simulink model "AC_Quadcopter_Simulation"  (R2019b)
settings: Solver=ode45  StartTime=0  StopTime=10  FixedStep=0.02  MaxStep=0.06  RelTol=1e-3  EnableMultiTasking=on
model workspace (MAT data in the model file):
  Sig = Simulink.Signal
  Sig.DataType = 'auto'
  Sig.Dimensions = -1
  Sig.DimensionsMode = 'auto'
  Sig.Complexity = 'auto'
  Sig.SampleTime = -1
  Sig.SamplingMode = 'auto'
undefined symbols (not defined in the file): IC, quadModel
libraries: simulink x4
Description:
  | This is a configurable quadcopter simulation.
  | This Simulink model demonstates attitude control.
  | 
  | Additional quadcopter modeling and simulation materials available at:
  | github.com/dch33/Quad-Sim
  | 
  | Copyright (C) 2014 D. Hartman, K. Landis, S. Moreno, J. Kim, M. Mehrer
  | 
  | License:
  |     This program is free software: you can redistribute it and/or modify
  |     it under the terms of the GNU LESSER GENERAL PUBLIC LICENSE as published by
  |     the Free Software Foundation, either version 3 of the License, or
  |     (at your option) any later version.
  | 
  |     This program is distributed in the hope that it will be useful,
  |     but WITHOUT ANY WARRANTY; without even the implied warranty of
  |     MERCHANTABILITY or FITNESS FOR A PARTICULAR PURPOSE.  See the
  |     GNU General Public License for more details.
  | 
  |     You should have received a copy of the GNU LESSER GENERAL PUBLIC LICENSE
  |     along with this program.  If not, see <http://www.gnu.org/licenses/>.
settings Model: ModifiedComment=davidhartman -- Fri Jun 06 23:19:51 2014 -- Version 1.5  Creator=David Hartman  LastModifiedBy=bhisma
settings Model: ModifiedHistory=|
  | davidhartman -- Fri Jun 06 23:19:51 2014 -- Version 1.5
  | 
  | 
  | davidhartman -- Fri Jun 06 23:19:51 2014 -- Version 1.5
  | 
  | 
  | davidhartman -- Fri Jun 06 22:53:10 2014 -- Version 1.3
settings SolverCC: AutoInsertRateTranBlk=on
settings DataIOCC: SaveFormat=Array  SignalLogging=off  ReturnWorkspaceOutputs=off
settings OptimizationCC: DefaultParameterBehavior=Inlined  LifeSpan=inf
settings DebuggingCC: UnderspecifiedInitializationDetection=Classic  MergeDetectMultiDrivingBlocksExec=none  SolverPrmCheckMsg=warning  UniqueDataStoreMsg=warning  StateNameClashWarn=warning  StrictBusMsg=WarnOnBusTreatedAsVector  SFUnexpectedBacktrackingDiag=warning  SFNoUnconditionalDefaultTransitionDiag=warning  SFExecutionAtInitializationDiag=none  ArithmeticOperatorsInVariantConditions=warning
settings HardwareCC: ProdBitPerPointer=32  ProdBitPerSizeT=32  ProdBitPerPtrDiffT=32  ProdLargestAtomicFloat=None  ProdIntDivRoundTo=Undefined  ProdEndianess=Unspecified  ProdWordSize=32  ProdHWDeviceType=32-bit Generic
settings ModelReferenceCC: PropagateSignalLabelsOutOfModel=off
settings SFSimCC: SimUseLocalCustomCode=off  CustomCodeUndefinedFunction=UseInterfaceOnly
settings RTWCC: RTWUseLocalCustomCode=off
settings CodeAppCC: StateflowObjectComments=on
settings GRTTargetCC: TargetLangStandard=C89/C90 (ANSI)  GeneratePreprocessorConditionals=Disable all
settings ConfigComp: CovMetricSettings=dw  CovHtmlReporting=on  CovSaveCumulativeToWorkspaceVar=on  CovSaveSingleToWorkspaceVar=on  CovExternalEMLEnable=off

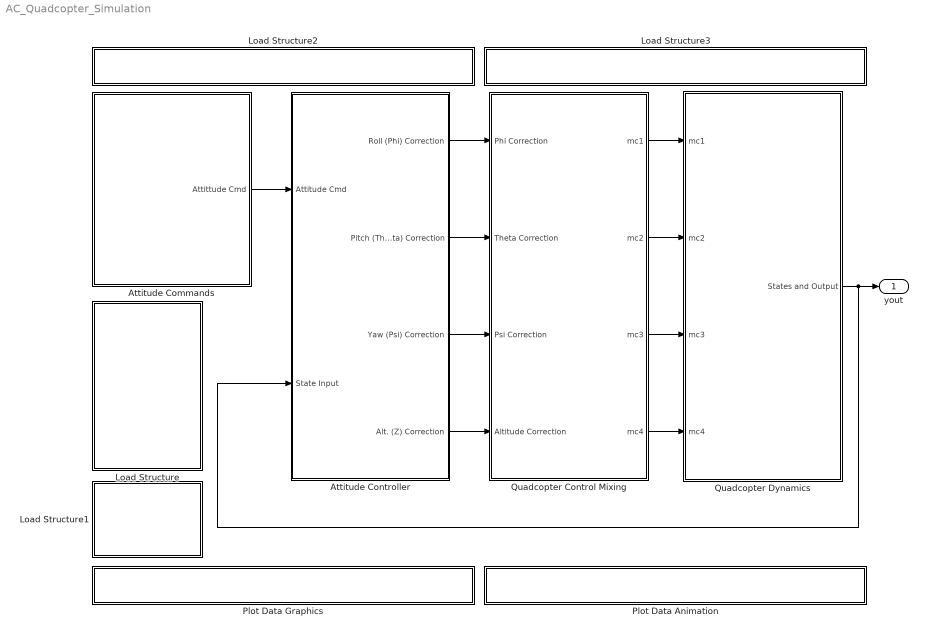
== system AC_Quadcopter_Simulation ==
  Attitude Commands : Subsystem
  Attitude Controller : Subsystem
  Load Structure : Subsystem
      settings: OpenFcn=|
      | uiopen('load')
      | if (exist('IC')==1 && exist('quadModel')==1)
      | set_param(bdroot, 'SimulationCommand', 'update')
      | end
      mask Display: fprintf('LOAD:\nQuadcopter\nModel Or\nInitial\nConditions');
  Load Structure1 : Subsystem
      settings: OpenFcn=|
      | if (exist('IC')==1 && exist('quadModel')==1 && exist('yout') && exist('tout'))
      | saveSimResults()
      | else
      | msgbox('No Data To Save!')
      | end
      mask Display: fprintf('SAVE:\nSimulation\nResults');
  Load Structure2 : Subsystem
      settings: OpenFcn=|
      | if exist('GUI_Modeling') == 2,
      | run('GUI_Modeling')
      | 
      | else
      | 
      | msgbox('The desired GUI must be first added to MATLABs path.')
      | 
      | end
      mask Display: fprintf('OPEN GUI: Build New \n Model');
  Load Structure3 : Subsystem
      settings: OpenFcn=|
      | if exist('GUI_IC') == 2,
      | run('GUI_IC')
      | 
      | else
      | 
      | msgbox('The desired GUI must be first added to MATLABs path.')
      | 
      | end
      mask Display: fprintf('OPEN GUI: Create Initial \n Conditions');
  Plot Data Animation : Subsystem
      settings: OpenFcn=|
      | if exist('QuadAnim4') == 2,
      |     if exist('yout')
      | 	run('QuadAnim4');
      |     else
      |     msgbox('Simulation must be run before data can be plotted.');
      |     end
      | else                                                                          msgbox('The desired GUI must be first added to MATLABs path.')
      | end
      mask Display: fprintf('OPEN GUI: Flight Animation')
  Plot Data Graphics : Subsystem
      settings: OpenFcn=|
      | if exist('yout')
      | yout = evalin('base', 'yout');
      | tout = evalin('base', 'tout');
      | quadPlots(yout, tout)
      | else
      | msgbox('Simulation must be run before data can be plotted.')
      | end
      mask Display: fprintf('OPEN PLOT: State Data')
  Quadcopter Control Mixing : Subsystem
      mask Display:
      | modelLoaded = evalin('base','exist(''quadModel'',''var'')');
      | if (modelLoaded==1)
      |     if (evalin('base','quadModel.plusConfig'))
      |     fprintf([' \n' ' \n'  'Configuration "+"']);
      |     else if (~evalin('base','quadModel.plusConfig'))
      |         fprintf([' \n' ' \n' 'Configuration "X"']);
      |         end
      |     end
      | else
      |     fprintf([' \n' ' \n'  'Model Not Loaded']);
      | end
  Quadcopter Dynamics : Subsystem
  yout : Outport
  wires:
  Quadcopter Dynamics/1(States and Output) -> yout/1, Attitude Controller/2(State Input)
  Quadcopter Control Mixing/1(mc1) -> Quadcopter Dynamics/1(mc1)
  Quadcopter Control Mixing/2(mc2) -> Quadcopter Dynamics/2(mc2)
  Quadcopter Control Mixing/3(mc3) -> Quadcopter Dynamics/3(mc3)
  Quadcopter Control Mixing/4(mc4) -> Quadcopter Dynamics/4(mc4)
  Attitude Controller/1(Roll (Phi) Correction) -> Quadcopter Control Mixing/1(Phi Correction)
  Attitude Controller/2(Pitch (Theta) Correction) -> Quadcopter Control Mixing/2(Theta Correction)
  Attitude Controller/3(Yaw (Psi) Correction) -> Quadcopter Control Mixing/3(Psi Correction)
  Attitude Controller/4(Alt. (Z) Correction) -> Quadcopter Control Mixing/4(Altitude Correction)
  Attitude Commands/1(Attittude Cmd) -> Attitude Controller/1(Attitude Cmd)

== system AC_Quadcopter_Simulation/Attitude Commands ==
  Bus Creator : BusCreator  Inputs=4
  Step : Step  Time=4  After=-10*pi/180  SampleTime=0
  Step1 : Step  After=10*pi/180  SampleTime=0
  Step2 : Step  Time=7  After=45*pi/180  SampleTime=0
  Step3 : Step  Time=0  Before=10*0.3048  After=10*0.3048  SampleTime=0
  Attittude Cmd : Outport
  tag scope: A=global
  wires:
  Bus Creator/1 -> Attittude Cmd/1, [A]  "Attitude_Cmd"
  Step3/1 -> Bus Creator/4  "Alt_cmd"
  Step2/1 -> Bus Creator/3  "Psi_cmd"
  Step1/1 -> Bus Creator/2  "The_cmd"
  Step/1 -> Bus Creator/1  "Phi_cmd"

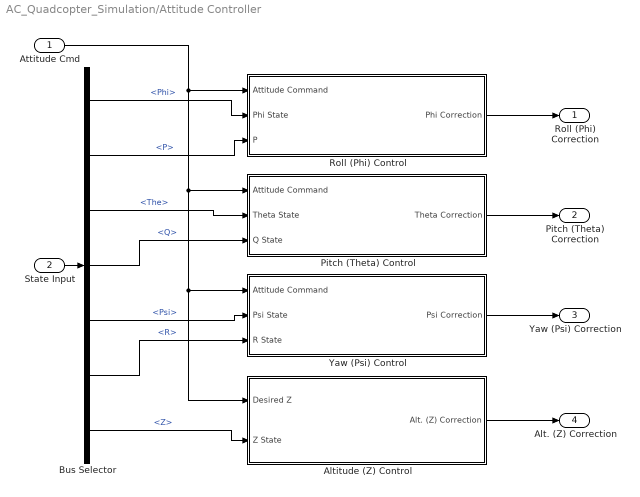
== system AC_Quadcopter_Simulation/Attitude Controller ==
  Attitude Cmd : Inport
  State Input : Inport  Port=2
  Altitude (Z) Control : Subsystem  mask{Kpz=2, Kiz=1.1, Kdz=3.3, LimitOutput=on, USat=1, LSat=-1, GOffset=(sqrt((quadModel.mass*quadModel.g)/(4*quadModel.ct))-quadModel.b)/quadModel.cr}
      mask prompts: Kpz "Kp"; Kiz "Ki"; Kdz "Kd"; LimitOutput "Integral Saturation?"; USat "Upper saturation limit:"; LSat "Lower saturation limit:"; GOffset "Gravity Feedforward"
      mask help:
      | Adjust PID controller gains through this mask interface, or "look under mask" for more detailed adjustments.
      |
      | Note: Gravity Offset will not appear on block face as a value until simulation is run if it is the result of a formula involving the quadcopter model parameters.
      mask TypeOptions Kpz: Kpz/Gain
      mask TypeOptions Kiz: Kiz/Gain
      mask TypeOptions Kdz: Kdz/Gain
      mask TypeOptions LimitOutput:
      | Integrator
      | Limited/LimitOutput
      mask TypeOptions USat:
      | Integrator
      | Limited/UpperSaturationLimit
      mask TypeOptions LSat:
      | Integrator
      | Limited/LowerSaturationLimit
      mask TypeOptions GOffset: Gravity Offset (Level Flight)/Value
      mask Display:
      | fprintf(['Gravity Offset = ' num2str(GOffset) '\n' ...
      |     'Kp = ' num2str(Kpz) '\n' ...
      |     'Ki = ' num2str(Kiz) '\n' ...
      |     'Kd = ' num2str(Kdz) '\n' ...
      |     'Integral Saturation: ' LimitOutput]);
      | if strcmp(LimitOutput,'on')
      |     fprintf([' \n' ' \n' ' \n' ' \n' ' \n' '\n' ...
      |         'Limits: ' num2str(USat) ' to ' num2str(LSat)]);
      | end
  Bus Selector : BusSelector  OutputSignals=Phi,P,The,Q,Psi,R,Z
  Pitch (Theta) Control : Subsystem  mask{Kpt=2, Kit=1.1, Kdt=1.2, LimitOutput=on, USat=1, LSat=-1}
      mask prompts: Kpt "Kp"; Kit "Ki"; Kdt "Kd"; LimitOutput "Integral Saturation?"; USat "Upper saturation limit:"; LSat "Lower saturation limit:"
      mask help: Adjust PID controller gains through this mask interface, or "look under mask" for more detailed adjustments.
      mask TypeOptions Kpt: Kpt/Gain
      mask TypeOptions Kit: Kit/Gain
      mask TypeOptions Kdt: Kdt/Gain
      mask TypeOptions LimitOutput:
      | Integrator
      | Limited/LimitOutput
      mask TypeOptions USat:
      | Integrator
      | Limited/UpperSaturationLimit
      mask TypeOptions LSat:
      | Integrator
      | Limited/LowerSaturationLimit
      mask Display:
      | fprintf(['Kp = ' num2str(Kpt) '\n' ...
      |     'Ki = ' num2str(Kit) '\n' ...
      |     'Kd = ' num2str(Kdt) '\n' ...
      |     'Integral Saturation: ' LimitOutput]);
      | if strcmp(LimitOutput,'on')
      |     fprintf([' \n' ' \n' ' \n' ' \n' '\n' ...
      |         'Limits: ' num2str(USat) ' to ' num2str(LSat)]);
      | end
  "Roll (Phi) Control " : Subsystem  mask{Kpp=2.0, Kip=1.1, Kdp=1.2, LimitOutput=on, USat=1, LSat=-1}
      mask prompts: Kpp "Kp"; Kip "Ki"; Kdp "Kd"; LimitOutput "Integral Saturation:"; USat "Upper saturation limit:"; LSat "Lower saturation limit:"
      mask help:
      | Adjust PID controller gains through this mask interface, or "look under mask"
      | for more detailed adjustments.
      mask TypeOptions Kpp: Kpp/Gain
      mask TypeOptions Kip: Kip/Gain
      mask TypeOptions Kdp: Kdp/Gain
      mask TypeOptions LimitOutput:
      | Integrator
      | Limited/LimitOutput
      mask TypeOptions USat:
      | Integrator
      | Limited/UpperSaturationLimit
      mask TypeOptions LSat:
      | Integrator
      | Limited/LowerSaturationLimit
      mask Display:
      | fprintf(['Kp = ' num2str(Kpp) '\n' ...
      |     'Ki = ' num2str(Kip) '\n' ...
      |     'Kd = ' num2str(Kdp) '\n'...
      |     'Integral Saturation: ' LimitOutput]);
      | if strcmp(LimitOutput,'on')
      |     fprintf([' \n' ' \n' ' \n' ' \n' '\n' ...
      |         'Limits: ' num2str(USat) ' to ' num2str(LSat)]);
      | end
  Yaw (Psi) Control : Subsystem  mask{Kps=4, Kis=0.5, Kds=3.5, LimitOutput=on, USat=1, LSat=-1}
      mask prompts: Kps "Kp"; Kis "Ki"; Kds "Kd"; LimitOutput "Integral Saturation?"; USat "Upper saturation limit:"; LSat "Lower saturation limit:"
      mask help: Adjust PID controller gains through this mask interface, or "look under mask" for more detailed adjustments.
      mask TypeOptions Kps: Kps/Gain
      mask TypeOptions Kis: Kit/Gain
      mask TypeOptions Kds: Kds/Gain
      mask TypeOptions LimitOutput:
      | Integrator
      | Limited/LimitOutput
      mask TypeOptions USat:
      | Integrator
      | Limited/UpperSaturationLimit
      mask TypeOptions LSat:
      | Integrator
      | Limited/LowerSaturationLimit
      mask Display:
      | fprintf(['Kp = ' num2str(Kps) '\n' ...
      |     'Ki = ' num2str(Kis) '\n' ...
      |     'Kd = ' num2str(Kds) '\n' ...
      |     'Integral Saturation: ' LimitOutput]);
      | if strcmp(LimitOutput,'on')
      |     fprintf([' \n' ' \n' ' \n' ' \n' '\n' ...
      |         'Limits: ' num2str(USat) ' to ' num2str(LSat)]);
      | end
  Roll (Phi) Correction : Outport
  Pitch (Theta) Correction : Outport  Port=2
  Yaw (Psi) Correction : Outport  Port=3
  Alt. (Z) Correction : Outport  Port=4
  wires:
  Bus Selector/6 -> Yaw (Psi) Control/3(R State)  "<R>"
  Bus Selector/4 -> Pitch (Theta) Control/3(Q State)  "<Q>"
  Bus Selector/2 -> "Roll (Phi) Control "/3(P)  "<P>"
  Bus Selector/3 -> Pitch (Theta) Control/2(Theta State)  "<The>"
  Attitude Cmd/1 -> "Roll (Phi) Control "/1("Attitude Command "), Pitch (Theta) Control/1(Attitude Command), Yaw (Psi) Control/1(Attitude Command), Altitude (Z) Control/1(Desired Z)
  Bus Selector/7 -> Altitude (Z) Control/2(Z State)  "<Z>"
  Altitude (Z) Control/1(Alt. (Z) Correction) -> Alt. (Z) Correction/1
  Bus Selector/5 -> Yaw (Psi) Control/2(Psi State)  "<Psi>"
  Yaw (Psi) Control/1(Psi Correction) -> Yaw (Psi) Correction/1
  Pitch (Theta) Control/1(Theta Correction) -> Pitch (Theta) Correction/1
  State Input/1 -> Bus Selector/1
  Bus Selector/1 -> "Roll (Phi) Control "/2(Phi State)  "<Phi>"
  "Roll (Phi) Control "/1(Phi Correction) -> Roll (Phi) Correction/1

== system AC_Quadcopter_Simulation/Load Structure ==

== system AC_Quadcopter_Simulation/Load Structure1 ==

== system AC_Quadcopter_Simulation/Load Structure2 ==

== system AC_Quadcopter_Simulation/Load Structure3 ==

== system AC_Quadcopter_Simulation/Plot Data Animation ==

== system AC_Quadcopter_Simulation/Plot Data Graphics ==

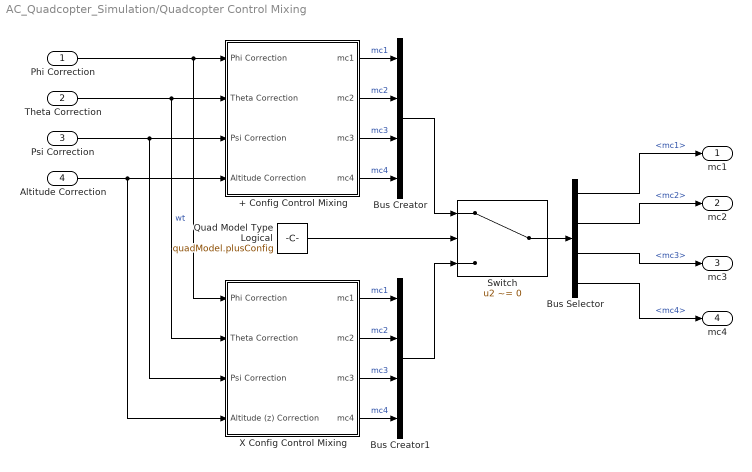
== system AC_Quadcopter_Simulation/Quadcopter Control Mixing ==
  Phi Correction : Inport
  Theta Correction : Inport  Port=2
  Psi Correction : Inport  Port=3
  Altitude Correction : Inport  Port=4
  + Config Control Mixing : Subsystem
  Bus Creator : BusCreator  Inputs=4
  Bus Creator1 : BusCreator  Inputs=4
  Bus Selector : BusSelector  OutputSignals=mc1,mc2,mc3,mc4
  Quad Model Type Logical : Constant  Value=quadModel.plusConfig
  Switch : Switch  Criteria=u2 ~= 0
  X Config Control Mixing : Subsystem
  mc1 : Outport
  mc2 : Outport  Port=2
  mc3 : Outport  Port=3
  mc4 : Outport  Port=4
  wires:
  Switch/1 -> Bus Selector/1
  Quad Model Type Logical/1 -> Switch/2
  Bus Selector/4 -> mc4/1  "<mc4>"
  Bus Selector/3 -> mc3/1  "<mc3>"
  Bus Selector/2 -> mc2/1  "<mc2>"
  Bus Selector/1 -> mc1/1  "<mc1>"
  Bus Creator1/1 -> Switch/3
  X Config Control Mixing/4(mc4) -> Bus Creator1/4  "mc4"
  X Config Control Mixing/3(mc3) -> Bus Creator1/3  "mc3"
  X Config Control Mixing/2(mc2) -> Bus Creator1/2  "mc2"
  X Config Control Mixing/1(mc1) -> Bus Creator1/1  "mc1"
  Bus Creator/1 -> Switch/1
  + Config Control Mixing/4(mc4) -> Bus Creator/4  "mc4"
  + Config Control Mixing/3(mc3) -> Bus Creator/3  "mc3"
  + Config Control Mixing/2(mc2) -> Bus Creator/2  "mc2"
  + Config Control Mixing/1(mc1) -> Bus Creator/1  "mc1"
  Altitude Correction/1 -> + Config Control Mixing/4(Altitude Correction), X Config Control Mixing/4(Altitude (z) Correction)
  Psi Correction/1 -> + Config Control Mixing/3(Psi Correction), X Config Control Mixing/3(Psi Correction)
  Theta Correction/1 -> + Config Control Mixing/2(Theta Correction), X Config Control Mixing/2(Theta Correction)  "wt"
  Phi Correction/1 -> + Config Control Mixing/1(Phi Correction), X Config Control Mixing/1(Phi Correction)

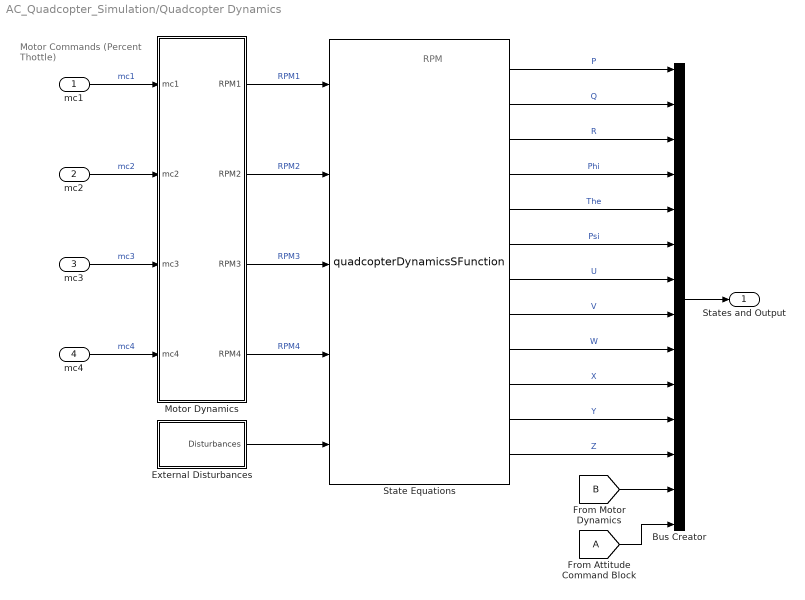
== system AC_Quadcopter_Simulation/Quadcopter Dynamics ==
  note: Motor Commands
      | (Percent Thottle)
  note: RPM
  mc1 : Inport
  mc2 : Inport  Port=2
  mc3 : Inport  Port=3
  mc4 : Inport  Port=4
  Bus Creator : BusCreator  Inputs='P','Q','R','Phi','The','Psi','U','V','W','X','Y','Z','mc and RPM','Attitude_Cmd'
  External Disturbances : Subsystem
  Motor Dynamics : Subsystem
  State Equations : M-S-Function  FunctionName=quadcopterDynamicsSFunction  Parameters=quadModel, IC
      mask Display:
      | port_label('input', 1, 'RPM1')
      | port_label('input', 2, 'RPM2')
      | port_label('input', 3, 'RPM3')
      | port_label('input', 4, 'RPM4')
      | port_label('input', 5, 'Disturbances')
      | port_label('output', 1, 'P')
      | port_label('output', 2, 'Q')
      | port_label('output', 3, 'R')
      | port_label('output', 4, 'Phi')
      | port_label('output', 5, 'The')
      | port_label('output', 6, 'Psi')
      | port_label('output', 7, 'U')
      | port_label('output', 8, 'V')
      | port_label('output', 9, 'W')
      | port_label('output', 10, 'X')
      | port_label('output', 11, 'Y')
      | port_label('output', 12, 'Z')
  States and Output : Outport
  wires:
  [B] -> Bus Creator/13
  [A] -> Bus Creator/14
  External Disturbances/1("Disturbances ") -> State Equations/5
  mc2/1 -> Motor Dynamics/2(mc2)  "mc2"
  mc3/1 -> Motor Dynamics/3(mc3)  "mc3"
  mc4/1 -> Motor Dynamics/4(mc4)  "mc4"
  mc1/1 -> Motor Dynamics/1(mc1)  "mc1"
  Motor Dynamics/4(RPM4) -> State Equations/4  "RPM4"
  Motor Dynamics/3(RPM3) -> State Equations/3  "RPM3"
  Motor Dynamics/2(RPM2) -> State Equations/2  "RPM2"
  Motor Dynamics/1(RPM1) -> State Equations/1  "RPM1"
  Bus Creator/1 -> States and Output/1
  State Equations/12 -> Bus Creator/12  "Z"
  State Equations/11 -> Bus Creator/11  "Y"
  State Equations/10 -> Bus Creator/10  "X"
  State Equations/9 -> Bus Creator/9  "W"
  State Equations/8 -> Bus Creator/8  "V"
  State Equations/7 -> Bus Creator/7  "U"
  State Equations/6 -> Bus Creator/6  "Psi"
  State Equations/5 -> Bus Creator/5  "The"
  State Equations/4 -> Bus Creator/4  "Phi"
  State Equations/3 -> Bus Creator/3  "R"
  State Equations/2 -> Bus Creator/2  "Q"
  State Equations/1 -> Bus Creator/1  "P"

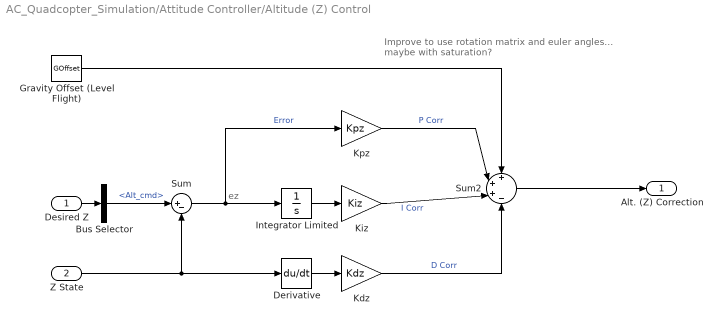
== system AC_Quadcopter_Simulation/Attitude Controller/Altitude (Z) Control ==
  note: ez
  note: Improve to use rotation matrix and euler angles...
      | maybe with saturation?
  Desired Z : Inport
  Z State : Inport  Port=2
  Bus Selector : BusSelector  OutputSignals=Alt_cmd
  Derivative : Derivative
  Gravity Offset (Level Flight) : Constant  Value=GOffset
  Integrator Limited : Integrator  LimitOutput=on  UpperSaturationLimit=USat  LowerSaturationLimit=LSat
  Kdz : Gain  Gain=Kdz
  Kiz : Gain  Gain=Kiz
  Kpz : Gain  Gain=Kpz
  Sum : Sum  Inputs=|+-
  Sum2 : Sum  Inputs=+++-
  Alt. (Z) Correction : Outport
  wires:
  Derivative/1 -> Kdz/1
  Bus Selector/1 -> Sum/1  "<Alt_cmd>"
  Integrator Limited/1 -> Kiz/1
  Kdz/1 -> Sum2/4  "D Corr"
  Kiz/1 -> Sum2/3  "I Corr"
  Sum/1 -> Kpz/1, Integrator Limited/1  "Error"
  Kpz/1 -> Sum2/2  "P Corr"
  Sum2/1 -> Alt. (Z) Correction/1
  Z State/1 -> Sum/2, Derivative/1
  Desired Z/1 -> Bus Selector/1
  Gravity Offset (Level Flight)/1 -> Sum2/1

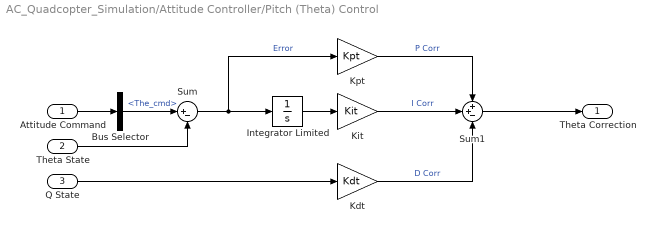
== system AC_Quadcopter_Simulation/Attitude Controller/Pitch (Theta) Control ==
  Attitude Command : Inport
  Theta State : Inport  Port=2
  Q State : Inport  Port=3
  Bus Selector : BusSelector  OutputSignals=The_cmd
  Integrator Limited : Integrator  LimitOutput=on  UpperSaturationLimit=USat  LowerSaturationLimit=LSat
  Kdt : Gain  Gain=Kdt
  Kit : Gain  Gain=Kit
  Kpt : Gain  Gain=Kpt
  Sum : Sum  Inputs=|+-
  Sum1 : Sum  Inputs=++-
  Theta Correction : Outport
  wires:
  Q State/1 -> Kdt/1
  Bus Selector/1 -> Sum/1  "<The_cmd>"
  Integrator Limited/1 -> Kit/1
  Kit/1 -> Sum1/2  "I Corr"
  Kdt/1 -> Sum1/3  "D Corr"
  Kpt/1 -> Sum1/1  "P Corr"
  Sum1/1 -> Theta Correction/1
  Theta State/1 -> Sum/2
  Attitude Command/1 -> Bus Selector/1
  Sum/1 -> Kpt/1, Integrator Limited/1  "Error"

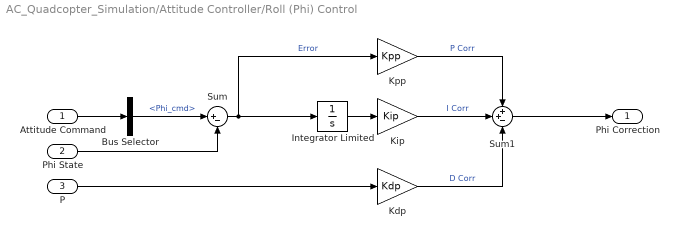
== system AC_Quadcopter_Simulation/Attitude Controller/Roll (Phi) Control  ==
  "Attitude Command " : Inport
  Phi State : Inport  Port=2
  P : Inport  Port=3
  Bus Selector : BusSelector  OutputSignals=Phi_cmd
  Integrator Limited : Integrator  LimitOutput=on  UpperSaturationLimit=USat  LowerSaturationLimit=LSat
  Kdp : Gain  Gain=Kdp
  Kip : Gain  Gain=Kip
  Kpp : Gain  Gain=Kpp
  Sum : Sum  Inputs=|+-
  Sum1 : Sum  Inputs=++-
  Phi Correction : Outport
  wires:
  P/1 -> Kdp/1
  Bus Selector/1 -> Sum/1  "<Phi_cmd>"
  "Attitude Command "/1 -> Bus Selector/1
  Integrator Limited/1 -> Kip/1
  Kip/1 -> Sum1/2  "I Corr"
  Kdp/1 -> Sum1/3  "D Corr"
  Kpp/1 -> Sum1/1  "P Corr"
  Sum1/1 -> Phi Correction/1
  Phi State/1 -> Sum/2
  Sum/1 -> Kpp/1, Integrator Limited/1  "Error"

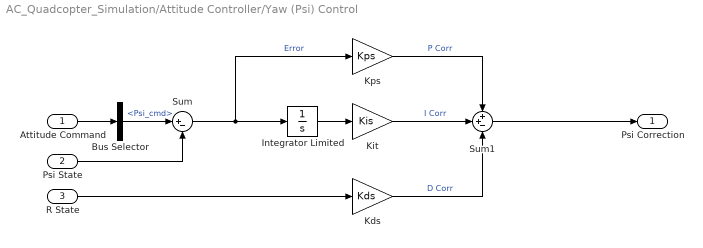
== system AC_Quadcopter_Simulation/Attitude Controller/Yaw (Psi) Control ==
  Attitude Command : Inport
  Psi State : Inport  Port=2
  R State : Inport  Port=3
  Bus Selector : BusSelector  OutputSignals=Psi_cmd
  Integrator Limited : Integrator  LimitOutput=on  UpperSaturationLimit=USat  LowerSaturationLimit=LSat
  Kds : Gain  Gain=Kds
  Kit : Gain  Gain=Kis
  Kps : Gain  Gain=Kps
  Sum : Sum  Inputs=|+-
  Sum1 : Sum  Inputs=++-
  Psi Correction : Outport
  wires:
  R State/1 -> Kds/1
  Bus Selector/1 -> Sum/1  "<Psi_cmd>"
  Integrator Limited/1 -> Kit/1
  Kit/1 -> Sum1/2  "I Corr"
  Kds/1 -> Sum1/3  "D Corr"
  Kps/1 -> Sum1/1  "P Corr"
  Psi State/1 -> Sum/2
  Sum1/1 -> Psi Correction/1
  Attitude Command/1 -> Bus Selector/1
  Sum/1 -> Kps/1, Integrator Limited/1  "Error"

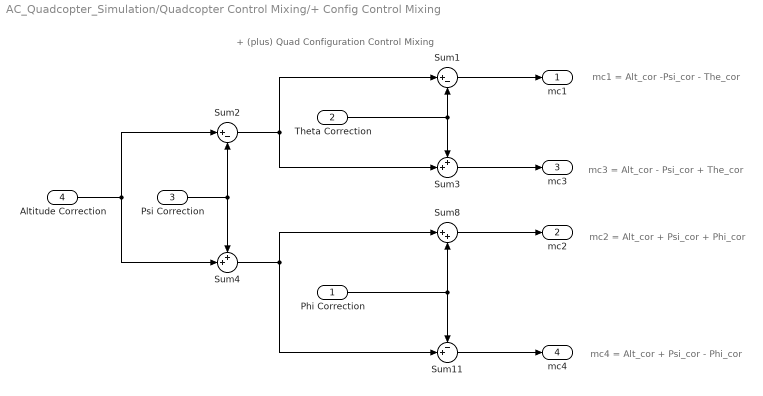
== system AC_Quadcopter_Simulation/Quadcopter Control Mixing/+ Config Control Mixing ==
  note: mc1 = Alt_cor -Psi_cor - The_cor
  note: mc3 = Alt_cor - Psi_cor + The_cor
  note: mc4 = Alt_cor + Psi_cor - Phi_cor
  note: + (plus) Quad Configuration Control Mixing
  note: mc2 = Alt_cor + Psi_cor + Phi_cor
  Phi Correction : Inport
  Theta Correction : Inport  Port=2
  Psi Correction : Inport  Port=3
  Altitude Correction : Inport  Port=4
  Sum1 : Sum  Inputs=|+-
  Sum11 : Sum  Inputs=-+|
  Sum2 : Sum  Inputs=|+-
  Sum3 : Sum  Inputs=++|
  Sum4 : Sum  Inputs=++|
  Sum8 : Sum  Inputs=|++
  mc1 : Outport
  mc2 : Outport  Port=2
  mc3 : Outport  Port=3
  mc4 : Outport  Port=4
  wires:
  Sum11/1 -> mc4/1
  Sum8/1 -> mc2/1
  Sum3/1 -> mc3/1
  Sum1/1 -> mc1/1
  Phi Correction/1 -> Sum11/1, Sum8/2
  Sum4/1 -> Sum8/1, Sum11/2
  Psi Correction/1 -> Sum2/2, Sum4/1
  Sum2/1 -> Sum1/1, Sum3/2
  Altitude Correction/1 -> Sum4/2, Sum2/1
  Theta Correction/1 -> Sum3/1, Sum1/2

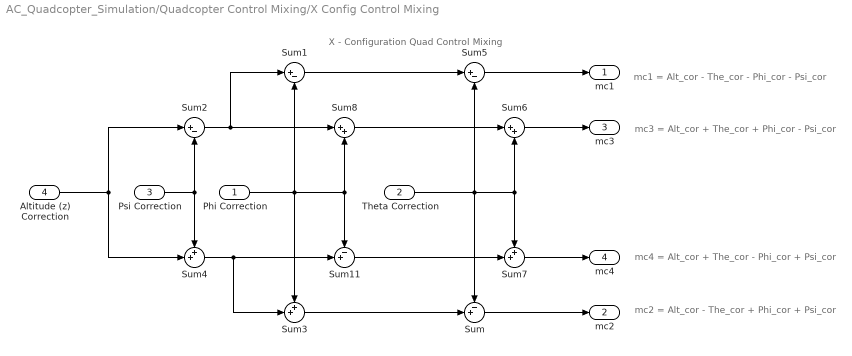
== system AC_Quadcopter_Simulation/Quadcopter Control Mixing/X Config Control Mixing ==
  note: mc4 = Alt_cor + The_cor - Phi_cor + Psi_cor
  note: mc2 = Alt_cor - The_cor + Phi_cor + Psi_cor
  note: mc3 = Alt_cor + The_cor + Phi_cor - Psi_cor
  note: X - Configuration Quad Control Mixing
  note: mc1 = Alt_cor - The_cor - Phi_cor - Psi_cor
  Phi Correction : Inport
  Theta Correction : Inport  Port=2
  Psi Correction : Inport  Port=3
  Altitude (z) Correction : Inport  Port=4
  Sum : Sum  Inputs=-+|
  Sum1 : Sum  Inputs=|+-
  Sum11 : Sum  Inputs=-+|
  Sum2 : Sum  Inputs=|+-
  Sum3 : Sum  Inputs=++|
  Sum4 : Sum  Inputs=++|
  Sum5 : Sum  Inputs=|+-
  Sum6 : Sum  Inputs=|++
  Sum7 : Sum  Inputs=++|
  Sum8 : Sum  Inputs=|++
  mc1 : Outport
  mc2 : Outport  Port=2
  mc3 : Outport  Port=3
  mc4 : Outport  Port=4
  wires:
  Sum/1 -> mc2/1
  Altitude (z) Correction/1 -> Sum4/2, Sum2/1
  Sum7/1 -> mc4/1
  Sum6/1 -> mc3/1
  Sum5/1 -> mc1/1
  Sum11/1 -> Sum7/2
  Sum8/1 -> Sum6/1
  Sum1/1 -> Sum5/1
  Theta Correction/1 -> Sum/1, Sum5/2, Sum6/2, Sum7/1
  Sum3/1 -> Sum/2
  Sum4/1 -> Sum11/2, Sum3/2
  Phi Correction/1 -> Sum11/1, Sum8/2, Sum1/2, Sum3/1
  Psi Correction/1 -> Sum2/2, Sum4/1
  Sum2/1 -> Sum1/1, Sum8/1

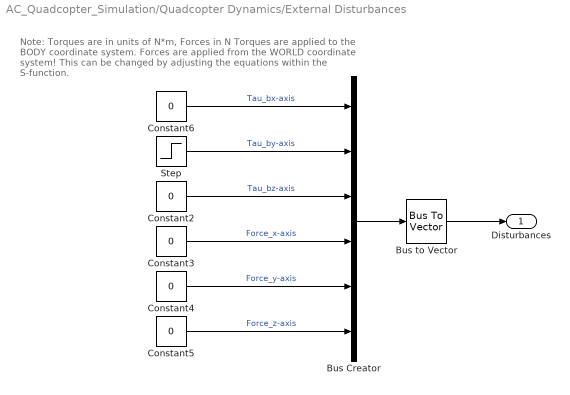
== system AC_Quadcopter_Simulation/Quadcopter Dynamics/External Disturbances ==
  note: Note: Torques are in units of N*m, Forces in N
      | Torques are applied to the BODY coordinate system.
      | Forces are applied from the WORLD coordinate system!
      | This can be changed by adjusting the equations within the S-function.
  Bus Creator : BusCreator  Inputs=6
  Bus to Vector : BusToVector
  Constant{2..6} (5 alike) : Constant  Value=0
  Step : Step  After=0  SampleTime=0
  "Disturbances " : Outport
  wires:
  Constant5/1 -> Bus Creator/6  "Force_z-axis"
  Constant4/1 -> Bus Creator/5  "Force_y-axis"
  Constant3/1 -> Bus Creator/4  "Force_x-axis"
  Constant2/1 -> Bus Creator/3  "Tau_bz-axis"
  Step/1 -> Bus Creator/2  "Tau_by-axis"
  Constant6/1 -> Bus Creator/1  "Tau_bx-axis"
  Bus Creator/1 -> Bus to Vector/1
  Bus to Vector/1 -> "Disturbances "/1

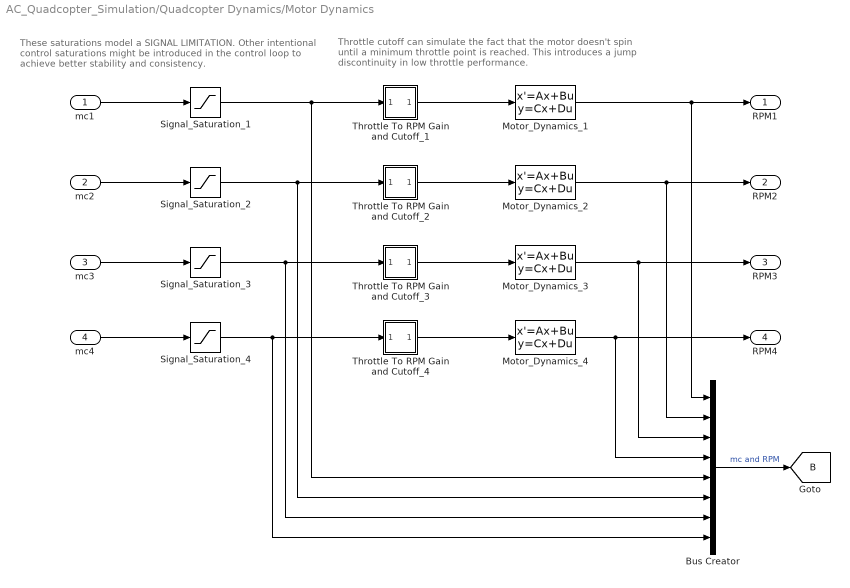
== system AC_Quadcopter_Simulation/Quadcopter Dynamics/Motor Dynamics ==
  note: These saturations model a SIGNAL LIMITATION.
      | Other intentional control saturations might be introduced in the
      | control loop to achieve better stability and consistency.
  note: Throttle cutoff can simulate the fact that the motor doesn't
      | spin until a minimum throttle point is reached. This introduces
      | a jump discontinuity in low throttle performance.
  mc1 : Inport
  mc2 : Inport  Port=2
  mc3 : Inport  Port=3
  mc4 : Inport  Port=4
  Bus Creator : BusCreator  Inputs=8
  Motor_Dynamics_1 : StateSpace  A=-1/quadModel.T  C=1/quadModel.T  D=0  InitialCondition=IC.w1*quadModel.T
  Motor_Dynamics_2 : StateSpace  A=-1/quadModel.T  C=1/quadModel.T  D=0  InitialCondition=IC.w2*quadModel.T
  Motor_Dynamics_3 : StateSpace  A=-1/quadModel.T  C=1/quadModel.T  D=0  InitialCondition=IC.w3*quadModel.T
  Motor_Dynamics_4 : StateSpace  A=-1/quadModel.T  C=1/quadModel.T  D=0  InitialCondition=IC.w4*quadModel.T
  Signal_Saturation_{1..4} (4 alike) : Saturate  UpperLimit=100  LowerLimit=0
  Throttle To RPM Gain and Cutoff_1 : Subsystem
  Throttle To RPM Gain and Cutoff_2 : Subsystem
  Throttle To RPM Gain and Cutoff_3 : Subsystem
  Throttle To RPM Gain and Cutoff_4 : Subsystem
  RPM1 : Outport
  RPM2 : Outport  Port=2
  RPM3 : Outport  Port=3
  RPM4 : Outport  Port=4
  tag scope: B=global
  wires:
  Bus Creator/1 -> [B]  "mc and RPM"
  Motor_Dynamics_4/1 -> RPM4/1, Bus Creator/4
  Motor_Dynamics_3/1 -> RPM3/1, Bus Creator/3
  Motor_Dynamics_2/1 -> RPM2/1, Bus Creator/2
  Motor_Dynamics_1/1 -> RPM1/1, Bus Creator/1
  Throttle To RPM Gain and Cutoff_4/1(Out5) -> Motor_Dynamics_4/1
  Throttle To RPM Gain and Cutoff_3/1(Out5) -> Motor_Dynamics_3/1
  Throttle To RPM Gain and Cutoff_2/1(Out5) -> Motor_Dynamics_2/1
  Throttle To RPM Gain and Cutoff_1/1(Out5) -> Motor_Dynamics_1/1
  Signal_Saturation_4/1 -> Throttle To RPM Gain and Cutoff_4/1(In5), Bus Creator/8
  Signal_Saturation_3/1 -> Throttle To RPM Gain and Cutoff_3/1(In5), Bus Creator/7
  Signal_Saturation_2/1 -> Throttle To RPM Gain and Cutoff_2/1(In5), Bus Creator/6
  Signal_Saturation_1/1 -> Throttle To RPM Gain and Cutoff_1/1(In5), Bus Creator/5
  mc3/1 -> Signal_Saturation_3/1
  mc2/1 -> Signal_Saturation_2/1
  mc4/1 -> Signal_Saturation_4/1
  mc1/1 -> Signal_Saturation_1/1

== system AC_Quadcopter_Simulation/Quadcopter Dynamics/Motor Dynamics/Throttle To RPM Gain and Cutoff_1 ==
  note: Output equals linearly scaled RPM
      | for given throttle input if throttle input >=Throttle Cuttoff (minThr)
      | else output is zero.
  In5 : Inport
  Constant : Constant  Value=quadModel.b
  Gain : Gain  Gain=quadModel.cr
  Minimum Throttle Cutoff : simulink/Logic and Bit Operations/Compare To Constant  relop=>=  const=quadModel.minThr  OutDataTypeStr=uint8
  Product : Product
  Sum1 : Sum  Inputs=++|
  Out5 : Outport
  wires:
  Constant/1 -> Sum1/1
  Sum1/1 -> Product/1
  Gain/1 -> Sum1/2
  In5/1 -> Minimum Throttle Cutoff/1, Gain/1
  Product/1 -> Out5/1
  Minimum Throttle Cutoff/1 -> Product/2

== system AC_Quadcopter_Simulation/Quadcopter Dynamics/Motor Dynamics/Throttle To RPM Gain and Cutoff_2 ==
  note: Output equals linearly scaled RPM
      | for given throttle input if throttle input >=Throttle Cuttoff (minThr)
      | else output is zero.
  In5 : Inport
  Constant : Constant  Value=quadModel.b
  Gain : Gain  Gain=quadModel.cr
  Minimum Throttle Cutoff : simulink/Logic and Bit Operations/Compare To Constant  relop=>=  const=quadModel.minThr  OutDataTypeStr=uint8
  Product : Product
  Sum1 : Sum  Inputs=++|
  Out5 : Outport
  wires:
  Constant/1 -> Sum1/1
  Sum1/1 -> Product/1
  Gain/1 -> Sum1/2
  In5/1 -> Minimum Throttle Cutoff/1, Gain/1
  Product/1 -> Out5/1
  Minimum Throttle Cutoff/1 -> Product/2

== system AC_Quadcopter_Simulation/Quadcopter Dynamics/Motor Dynamics/Throttle To RPM Gain and Cutoff_3 ==
  note: Output equals linearly scaled RPM
      | for given throttle input if throttle input >=Throttle Cuttoff (minThr)
      | else output is zero.
  In5 : Inport
  Constant : Constant  Value=quadModel.b
  Gain : Gain  Gain=quadModel.cr
  Minimum Throttle Cutoff : simulink/Logic and Bit Operations/Compare To Constant  relop=>=  const=quadModel.minThr  OutDataTypeStr=uint8
  Product : Product
  Sum1 : Sum  Inputs=++|
  Out5 : Outport
  wires:
  Constant/1 -> Sum1/1
  Sum1/1 -> Product/1
  Gain/1 -> Sum1/2
  In5/1 -> Minimum Throttle Cutoff/1, Gain/1
  Product/1 -> Out5/1
  Minimum Throttle Cutoff/1 -> Product/2

== system AC_Quadcopter_Simulation/Quadcopter Dynamics/Motor Dynamics/Throttle To RPM Gain and Cutoff_4 ==
  note: Output equals linearly scaled RPM
      | for given throttle input if throttle input >=Throttle Cuttoff (minThr)
      | else output is zero.
  In5 : Inport
  Constant : Constant  Value=quadModel.b
  Gain : Gain  Gain=quadModel.cr
  Minimum Throttle Cutoff : simulink/Logic and Bit Operations/Compare To Constant  relop=>=  const=quadModel.minThr  OutDataTypeStr=uint8
  Product : Product
  Sum1 : Sum  Inputs=++|
  Out5 : Outport
  wires:
  Constant/1 -> Sum1/1
  Sum1/1 -> Product/1
  Gain/1 -> Sum1/2
  In5/1 -> Minimum Throttle Cutoff/1, Gain/1
  Product/1 -> Out5/1
  Minimum Throttle Cutoff/1 -> Product/2
